simulink model "simu_6b"  (R2015a)
settings: Solver=ode45  StartTime=0.0  StopTime=10.0  RelTol=1e-3
settings Model: Creator=Aluno-05  LastModifiedBy=Aluno-05

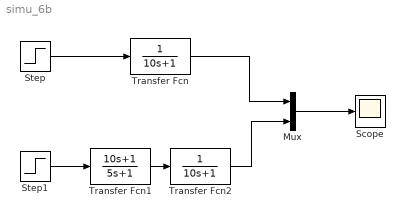
== system simu_6b ==
  Mux : Mux  Inputs=2
  Scope : Scope
  Step : Step  SampleTime=0
  Step1 : Step  SampleTime=0
  Transfer Fcn : TransferFcn  Denominator=[10 1]
  Transfer Fcn1 : TransferFcn  Numerator=[10 1]  Denominator=[5 1]
  Transfer Fcn2 : TransferFcn  Denominator=[10 1]
  wires:
  Step/1 -> Transfer Fcn/1
  Transfer Fcn/1 -> Mux/1
  Step1/1 -> Transfer Fcn1/1
  Mux/1 -> Scope/1
  Transfer Fcn1/1 -> Transfer Fcn2/1
  Transfer Fcn2/1 -> Mux/2
